simulink model "SimulationEnvironment"  (R2019b)
settings: Solver=VariableStepAuto  StartTime=0.0  StopTime=10.0  RelTol=1e-3
settings Model: Creator=loker  LastModifiedBy=lgt9489

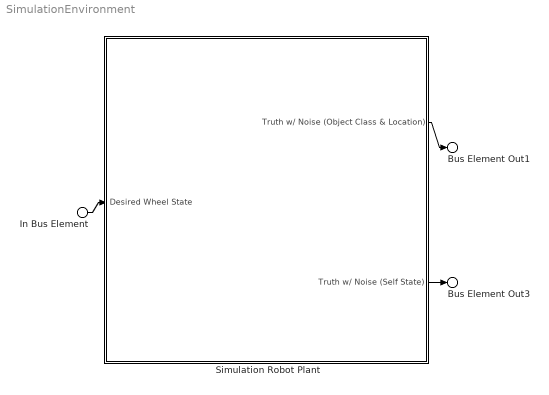
== system SimulationEnvironment ==
  In Bus Element : Inport  PortName=Desired Wheel State
  Simulation Robot Plant : Subsystem
      settings: PortSchema="{\"entries\":[{\"content\":{\"headerSize\":26,\"margin\":15,\"minimumSpacing\":25,\"sides\":[{\"content\":{\"connectorIds\":[\"In1\"]},\"type\":\"ConnectorPlacement.EquallySpacedRectSide\",\"uuid\":\"9c658e47-9141-4b09-899d-e7d6eeef288e\"},{\"content\":{\"connectorIds\":[\"Out1\",\"Out2\"],\"side\":\"RIGHT\"},\"type\":\"ConnectorPlacement.EquallySpacedRectSide\",\"uuid\":\"7a582264-0565-42d4-adb3-e560ad597e55\"},{\"content\":{\"connectorIds\":[],\"side\":\"TOP\"},\"type\":\"ConnectorPlacement.EquallySpacedRectSide\",\"uuid\":\"701b4c6c-e203-4bd7-b8b7-cb8feb01699c\"},{\"content\":{\"connectorIds\":[],\"side\":\"BOTTOM\"},\"type\":\"ConnectorPlacement.EquallySpacedRectSide\",\"uuid\":\"cabe974f-2bf0-4fd9-b8de-04e88f14bcad\"}]},\"type\":\"ConnectorPlacement.EquallySpacedConnector\",\"uuid\":\"2059a5e9-c0d5-4fb6-87cf-b1bfdc666ab8\"}],\"packageUris\":[\"http://schema.mathworks.com/mf0/Connector/19700101\"],\"version\":\"1.0\"}"
  Bus Element Out1 : Outport  PortName=Truth w/ Noise (Object Class & Location)
  Bus Element Out3 : Outport  Port=2  PortName=Truth w/ Noise (Self State)
  wires:
  Simulation Robot Plant/1(Truth w/ Noise (Object Class & Location)) -> Bus Element Out1/1
  Simulation Robot Plant/2(Truth w/ Noise (Self State)) -> Bus Element Out3/1
  In Bus Element/1 -> Simulation Robot Plant/1(Desired Wheel State)

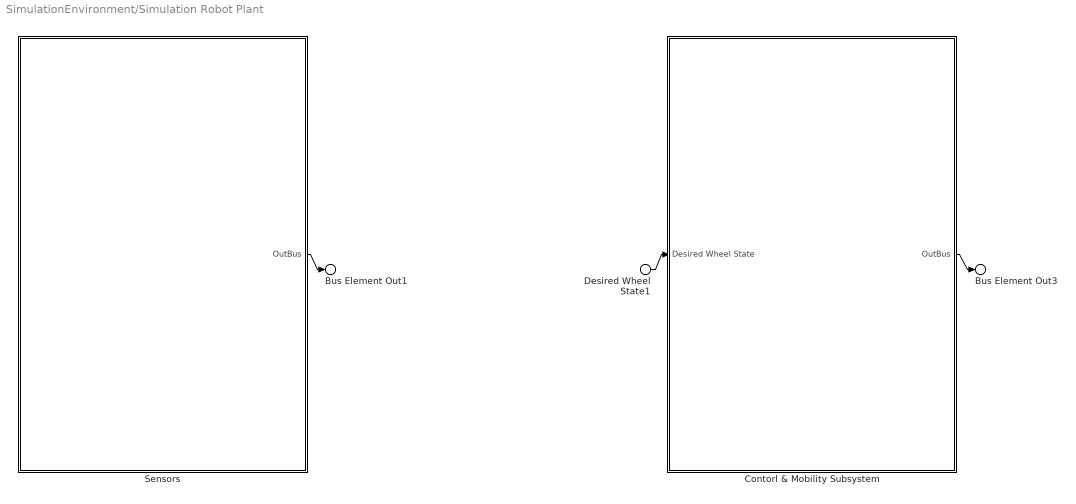
== system SimulationEnvironment/Simulation Robot Plant ==
  Desired Wheel State1 : Inport  PortName=Desired Wheel State
  Contorl & Mobility Subsystem : Subsystem
      settings: PortSchema="{\"entries\":[{\"content\":{\"headerSize\":26,\"margin\":15,\"minimumSpacing\":25,\"sides\":[{\"content\":{\"connectorIds\":[\"In1\"]},\"type\":\"ConnectorPlacement.EquallySpacedRectSide\",\"uuid\":\"9c658e47-9141-4b09-899d-e7d6eeef288e\"},{\"content\":{\"connectorIds\":[\"Out1\"],\"side\":\"RIGHT\"},\"type\":\"ConnectorPlacement.EquallySpacedRectSide\",\"uuid\":\"7a582264-0565-42d4-adb3-e560ad597e55\"},{\"content\":{\"connectorIds\":[],\"side\":\"TOP\"},\"type\":\"ConnectorPlacement.EquallySpacedRectSide\",\"uuid\":\"701b4c6c-e203-4bd7-b8b7-cb8feb01699c\"}]},\"type\":\"ConnectorPlacement.EquallySpacedConnector\",\"uuid\":\"2059a5e9-c0d5-4fb6-87cf-b1bfdc666ab8\"}],\"packageUris\":[\"http://schema.mathworks.com/mf0/Connector/19700101\"],\"version\":\"1.0\"}"
  Sensors : Subsystem
      settings: PortSchema="{\"entries\":[{\"content\":{\"headerSize\":26,\"margin\":15,\"minimumSpacing\":25,\"sides\":[{\"content\":{\"connectorIds\":[]},\"type\":\"ConnectorPlacement.EquallySpacedRectSide\",\"uuid\":\"1e9d356f-7e7b-426d-8d98-f3c7def5de5c\"},{\"content\":{\"connectorIds\":[\"Out1\"],\"side\":\"RIGHT\"},\"type\":\"ConnectorPlacement.EquallySpacedRectSide\",\"uuid\":\"0e4583bd-4f23-4fa6-8e05-59fd9be96908\"},{\"content\":{\"connectorIds\":[],\"side\":\"TOP\"},\"type\":\"ConnectorPlacement.EquallySpacedRectSide\",\"uuid\":\"d7ab4f72-14a0-4c6c-a9cc-bd21825fdf14\"}]},\"type\":\"ConnectorPlacement.EquallySpacedConnector\",\"uuid\":\"d1e9dbce-5e63-4c1c-8863-79e46a312bbf\"}],\"packageUris\":[\"http://schema.mathworks.com/mf0/Connector/19700101\"],\"version\":\"1.0\"}"
  Bus Element Out1 : Outport  PortName=Truth w/ Noise (Object Class & Location)
  Bus Element Out3 : Outport  Port=2  PortName=Truth w/ Noise (Self State)
  wires:
  Desired Wheel State1/1 -> Contorl & Mobility Subsystem/1(Desired Wheel State)
  Sensors/1(OutBus) -> Bus Element Out1/1
  Contorl & Mobility Subsystem/1(OutBus) -> Bus Element Out3/1

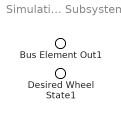
== system SimulationEnvironment/Simulation Robot Plant/Contorl & Mobility Subsystem ==
  Desired Wheel State1 : Inport  PortName=Desired Wheel State
  Bus Element Out1 : Outport  PortName=OutBus

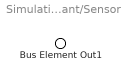
== system SimulationEnvironment/Simulation Robot Plant/Sensors ==
  Bus Element Out1 : Outport  PortName=OutBus
